simulink model "MATLAB Simulink Model"  (R2020b)
settings: Solver=ode4  StartTime=0.0  StopTime=1  RelTol=1e-3
InitFcn:
  | clear;
  | clc;
  | 
  | %Motor Parameters
  | r1 = 1.405;
  | l1  = 0.005839;
  | r2 = 1.395;
  | l2 = 0.005839;
  | Lm = 0.1722;
  | 
  | %Motor Rated Values
  | Vrat = 400;
  | frat = 50;
  | 
  | x1 = 2*pi*frat*l1;
  | x2 = 2*pi*frat*l2;
  | Xm = 2*pi*frat*Lm;
  | Prat = 4*1000;
  | Nrat = 1430;
  | Ns = 120*frat/4;
  | nrat = Nrat*2*pi/60;
  | ns = Ns*2*pi/60;
  | srat = (Ns-Nrat)/Ns;
  | 
  | E1 = Vrat/sqrt(3); %phase voltage
  | IL = E1/( (r1 + (1i*x1) ) + ( ( (1i*x2) +(r2/srat) )*1i*Xm / ( (1i*Xm) + (1i*x2) + (r2/srat) ) ) );
  | E2 = E1 - (IL*(r1 + (1i*x1) ) );
  | Trat = (3/(ns))*srat*abs(E2)*abs(E2)*r2/((r2*r2) + (srat*srat*x2*x2));
  | %Trat = Prat/nrat;
  | 
  | %System Variables
  | Tsys = (1e-6);
  | Ts = (100e-6);
  | freq = 50;
  | 
  | m=1*freq/50;
  | %m = 1 * (freq/50);
  | Vbus = (400*sqrt(2)*2/sqrt(3)) / (1.15);
  | 
  | Vref = (Vbus*sqrt(3)/2) * m;
  | delay = Ts/Tsys;
  | 
  | % Motor Starting Parameters
  | inc_time = 0.1;
  | 
  | %Motor Loading time
  | load_time = 0.5;
  | 
  | %No. of Hybrid Zones
  | numzones = 3;
  | 
  | %Load ML model Weights
  | 
  | W1R_s1 = readmatrix('Regression Weights\W1_subnet1_tmp_odd_90.xlsx');
  | b1R_s1 = readmatrix('Regression Weights\b1_subnet1_tmp_odd_90.xlsx');
  | W1R_s2 = readmatrix('Regression Weights\W1_subnet2_tmp_odd_90.xlsx');
  | b1R_s2 = readmatrix('Regression Weights\b1_subnet2_tmp_odd_90.xlsx');
  | 
  | W2R = readmatrix('Regression Weights\W2_subnet_tmp_odd_90.xlsx');
  | b2R = readmatrix('Regression Weights\b2_subnet_tmp_odd_90.xlsx');
  | ... (+9 lines)
libraries: powerlib x72, simulink x55, powerlib_meascontrol x15, dspstat3 x11, dspsigops x1
(part 5 of 5)

== matlab function MATLAB Simulink Model/Space Vector PWM based VSI /Switching Times and Sector/Feature Expand1 ==
  data: X input; new_X output size=[1 90]
function new_X = fcn(X)
    X = X';
    new_X = zeros(1,90);
    new_X(1, 1) = X(1, 1);
    new_X(1, 2) = X(1, 2);
    
    %Include sinusoidal terms (1st order)
    new_X(1, 3) = sin(X(1, 1));
    new_X(1, 4) = sin(X(1, 2));
    new_X(1, 5) = cos(X(1, 1));
    new_X(1, 6) = cos(X(1, 2));
%     new_X(1, 7) = sin(X(1, 1).*X(1, 2));
%     new_X(1, 8) = cos(X(1, 1).*X(1, 2));
    
% %Include 2nd harmonic sinusoidal terms
%     new_X(1, 7) = sin(2*X(1, 1));
%     new_X(1, 8) = sin(2*X(1, 2));
%     new_X(1, 9) = cos(2*X(1, 1));
%     new_X(1, 10) = cos(2*X(1, 2));
    
        %Include 3rd harmonic sinusoidal terms
    new_X(1, 7) = sin(3*X(1, 1));
    new_X(1, 8) = sin(3*X(1, 2));
    new_X(1, 9) = cos(3*X(1, 1));
    new_X(1, 10) = cos(3*X(1, 2));
    
%     %Include 4th harmonic sinusoidal terms
%     new_X(1, 15) = sin(4*X(1, 1));
%     new_X(1, 16) = sin(4*X(1, 2));
%     new_X(1, 17) = cos(4*X(1, 1));
%     new_X(1, 18) = cos(4*X(1, 2));
       %Include 5th harmonic sinusoidal terms
    new_X(1, 11) = sin(5*X(1, 1));
    new_X(1, 12) = sin(5*X(1, 2));
    new_X(1, 13) = cos(5*X(1, 1));
    new_X(1, 14) = cos(5*X(1, 2));
    
       %Include 7th harmonic sinusoidal terms
    new_X(1, 15) = sin(7*X(1, 1));
    new_X(1, 16) = sin(7*X(1, 2));
    new_X(1, 17) = cos(7*X(1, 1));
    new_X(1, 18) = cos(7*X(1, 2));
    
       %Include 9th harmonic sinusoidal terms
    new_X(1, 19) = sin(9*X(1, 1));
    new_X(1, 20) = sin(9*X(1, 2));
    new_X(1, 21) = cos(9*X(1, 1));
    new_X(1, 22) = cos(9*X(1, 2));

       %Include 11th harmonic sinusoidal terms
    new_X(1, 23) = sin(11*X(1, 1));
    new_X(1, 24) = sin(11*X(1, 2));
    new_X(1, 25) = cos(11*X(1, 1));
    new_X(1, 26) = cos(11*X(1, 2));
    
         %Include 13th harmonic sinusoidal terms
    new_X(1, 27) = sin(13*X(1, 1));
    new_X(1, 28) = sin(13*X(1, 2));
    new_X(1, 29) = cos(13*X(1, 1));
    new_X(1, 30) = cos(13*X(1, 2));
    
         %Include 15th harmonic sinusoidal terms
    new_X(1, 31) = sin(15*X(1, 1));
    new_X(1, 32) = sin(15*X(1, 2));
    new_X(1, 33) = cos(15*X(1, 1));
    new_X(1, 34) = cos(15*X(1, 2));
    
    %Include 17th harmonic sinusoidal terms
    new_X(1, 35) = sin(17*X(1, 1));
    new_X(1, 36) = sin(17*X(1, 2));
    new_X(1, 37) = cos(17*X(1, 1));
    new_X(1, 38) = cos(17*X(1, 2));
    
    %Include 19th harmonic sinusoidal terms
    new_X(1, 39) = sin(19*X(1, 1));
    new_X(1, 40) = sin(19*X(1, 2));
    new_X(1, 41) = cos(19*X(1, 1));
    new_X(1, 42) = cos(19*X(1, 2));
    
    %Include 21th harmonic sinusoidal terms
    new_X(1, 43) = sin(21*X(1, 1));
    new_X(1, 44) = sin(21*X(1, 2));
    new_X(1, 45) = cos(21*X(1, 1));
    new_X(1, 46) = cos(21*X(1, 2));
    
    %Include 23th harmonic sinusoidal terms
    new_X(1, 47) = sin(23*X(1, 1));
    new_X(1, 48) = sin(23*X(1, 2));
    new_X(1, 49) = cos(23*X(1, 1));
    new_X(1, 50) = cos(23*X(1, 2));

    %Include 25th harmonic sinusoidal terms
    new_X(1, 51) = sin(25*X(1, 1));
    new_X(1, 52) = sin(25*X(1, 2));
    new_X(1, 53) = cos(25*X(1, 1));
    new_X(1, 54) = cos(25*X(1, 2));

%Include 27th harmonic sinusoidal terms
    new_X(1, 55) = sin(27*X(1, 1));
    new_X(1, 56) = sin(27*X(1, 2));
    new_X(1, 57) = cos(27*X(1, 1));
    new_X(1, 58) = cos(27*X(1, 2));
    
%Include 29th harmonic sinusoidal terms
    new_X(1, 59) = sin(29*X(1, 1));
    new_X(1, 60) = sin(29*X(1, 2));
    new_X(1, 61) = cos(29*X(1, 1));
    new_X(1, 62) = cos(29*X(1, 2));

%Include 31th harmonic sinusoidal terms
    new_X(1, 63) = sin(31*X(1, 1));
    new_X(1, 64) = sin(31*X(1, 2));
    new_X(1, 65) = cos(31*X(1, 1));
    new_X(1, 66) = cos(31*X(1, 2));

%Include 33th harmonic sinusoidal terms
    new_X(1, 67) = sin(33*X(1, 1));
    new_X(1, 68) = sin(33*X(1, 2));
    new_X(1, 69) = cos(33*X(1, 1));
    new_X(1, 70) = cos(33*X(1, 2));
    
%Include 35th harmonic sinusoidal terms
    new_X(1, 71) = sin(35*X(1, 1));
    new_X(1, 72) = sin(35*X(1, 2));
    new_X(1, 73) = cos(35*X(1, 1));
    new_X(1, 74) = cos(35*X(1, 2));
    
%Include 37th harmonic sinusoidal terms
    new_X(1, 75) = sin(37*X(1, 1));
    new_X(1, 76) = sin(37*X(1, 2));
    new_X(1, 77) = cos(37*X(1, 1));
    new_X(1, 78) = cos(37*X(1, 2));
    
%Include 39th harmonic sinusoidal terms
    new_X(1, 79) = sin(39*X(1, 1));
    new_X(1, 80) = sin(39*X(1, 2));
    new_X(1, 81) = cos(39*X(1, 1));
    new_X(1, 82) = cos(39*X(1, 2));
    
%Include 41th harmonic sinusoidal terms
    new_X(1, 83) = sin(41*X(1, 1));
    new_X(1, 84) = sin(41*X(1, 2));
    new_X(1, 85) = cos(41*X(1, 1));
    new_X(1, 86) = cos(41*X(1, 2));

%Include 43th harmonic sinusoidal terms
    new_X(1, 87) = sin(43*X(1, 1));
    new_X(1, 88) = sin(43*X(1, 2));
    new_X(1, 89) = cos(43*X(1, 1));
    new_X(1, 90) = cos(43*X(1, 2));
%     %Include 2nd order terms
%     new_X(:, 3) = X(:, 1).*X(:, 1);
%     new_X(:, 4) = X(:, 1).*X(:, 2);
%     new_X(:, 5) = X(:, 2).*X(:, 2);
    
%     %Include 3rd order terms
%     new_X(:, 6) = X(:, 1).*X(:, 1).*X(:, 1);
%     new_X(:, 7) = X(:, 1).*X(:, 1).*X(:, 2);
%     new_X(:, 8) = X(:, 1).*X(:, 2).*X(:, 2);
%     new_X(:, 9) = X(:, 2).*X(:, 2).*X(:, 2);
%     
%     %Incluce 4th order terms
%     new_X(:, 10) = X(:, 1).*X(:, 1).*X(:, 1).*X(:, 1);
%     new_X(:, 11) = X(:, 1).*X(:, 1).*X(:, 1).*X(:, 2);
%     new_X(:, 12) = X(:, 1).*X(:, 1).*X(:, 2).*X(:, 2);
%     new_X(:, 13) = X(:, 1).*X(:, 2).*X(:, 2).*X(:, 2);
%     new_X(:, 14) = X(:, 2).*X(:, 2).*X(:, 2).*X(:, 2);
%     
%     %Incluce 5th order terms
%     new_X(:, 15) = X(:, 1).*X(:, 1).*X(:, 1).*X(:, 1).*X(:, 1);
%     new_X(:, 16) = X(:, 1).*X(:, 1).*X(:, 1).*X(:, 1).*X(:, 2);
%     new_X(:, 17) = X(:, 1).*X(:, 1).*X(:, 1).*X(:, 2).*X(:, 2);
%     new_X(:, 18) = X(:, 1).*X(:, 1).*X(:, 2).*X(:, 2).*X(:, 2);
%     new_X(:, 19) = X(:, 1).*X(:, 2).*X(:, 2).*X(:, 2).*X(:, 2);
%     new_X(:, 20) = X(:, 2).*X(:, 2).*X(:, 2).*X(:, 2).*X(:, 2);
%     
%     %Incluce 6th order terms
%     new_X(:, 21) = X(:, 1).*X(:, 1).*X(:, 1).*X(:, 1).*X(:, 1).*X(:, 1);
%     new_X(:, 22) = X(:, 1).*X(:, 1).*X(:, 1).*X(:, 1).*X(:, 1).*X(:, 2);
%     new_X(:, 23) = X(:, 1).*X(:, 1).*X(:, 1).*X(:, 1).*X(:, 2).*X(:, 2);
%     new_X(:, 24) = X(:, 1).*X(:, 1).*X(:, 1).*X(:, 2).*X(:, 2).*X(:, 2);
%     new_X(:, 25) = X(:, 1).*X(:, 1).*X(:, 2).*X(:, 2).*X(:, 2).*X(:, 2);
%     new_X(:, 26) = X(:, 1).*X(:, 2).*X(:, 2).*X(:, 2).*X(:, 2).*X(:, 2);
%     new_X(:, 27) = X(:, 2).*X(:, 2).*X(:, 2).*X(:, 2).*X(:, 2).*X(:, 2);
end

== matlab function MATLAB Simulink Model/Space Vector PWM based VSI /Switching Times and Sector/MATLAB Function ==
  data: u input; y output
function y = fcn(u)
    y = 1./(1+exp(-1*u));
end

== matlab function MATLAB Simulink Model/RMS Error Calculation /Subsystem/MATLAB Function1 ==
  data: Tsys input; Ts input; phi_q input; phi_q_rms input; prev_it_num input; phi_q_rms output; curr_it_num output
function [phi_q_rms, curr_it_num]= fcn( Tsys, Ts, phi_q, phi_q_rms, prev_it_num)
curr_it_num = prev_it_num+1;

if  int16(curr_it_num) == int16(Ts/Tsys)
    phi_q_rms=0;
    curr_it_num = 1;
end

phi_q_rms = phi_q_rms + (abs(phi_q)*abs(phi_q)*Tsys);
end

== matlab function MATLAB Simulink Model/3 Phase Induction Machine1/Angle Calculation/MATLAB Function ==
  data: wold input; wnew output; wTs input
function wnew = fcn(wold, wTs)
    wnew = rem(wold + wTs, 2*pi);
end

== matlab function MATLAB Simulink Model/3 Phase Induction Machine1/MATLAB Function ==
  data: phi_d input; T_calc output; phi_q input; i_d input; i_q input
function T_calc = fcn(phi_d, phi_q, i_d, i_q)
    phi_s = phi_d + (1i*phi_q);
    i_s = i_d + (1i*i_q);
    T_calc = (-3)*real(1i*phi_s * i_s);
end

== matlab function MATLAB Simulink Model/3 Phase Induction Machine/MATLAB Function ==
  data: phi_d input; T_calc output; phi_q input; i_d input; i_q input
function T_calc = fcn(phi_d, phi_q, i_d, i_q)
    phi_s = phi_d + (1i*phi_q);
    i_s = i_d + (1i*i_q);
    T_calc = (-3)*real(1i*phi_s * i_s);
end
